simulink model "DC_Microgrid_Protection"  (R2022a)
settings: Solver=ode4  StartTime=0.0  StopTime=10  FixedStep=0.01  RelTol=1e-3
settings Model: Creator=nivas  LastModifiedBy=nivas

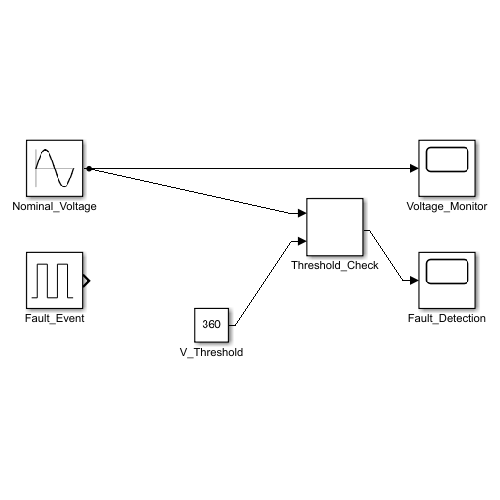
[thumbnail: Simulink's stored preview of the top-level diagram]
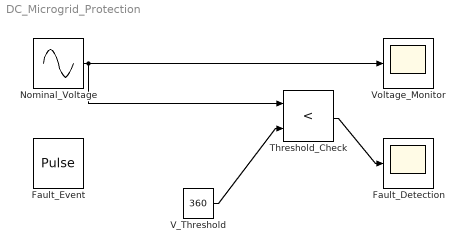
== system DC_Microgrid_Protection ==
  Fault_Detection : Scope
  Fault_Event : DiscretePulseGenerator  PulseType=Time based  Period=5  PulseWidth=20
  Nominal_Voltage : Sin  Amplitude=10  Bias=400  Frequency=0.5  SampleTime=0
  Threshold_Check : RelationalOperator  Operator=<  OutDataTypeStr=boolean  RndMeth=Simplest  InputSameDT=off
  V_Threshold : Constant  Value=360
  Voltage_Monitor : Scope
  wires:
  Nominal_Voltage/1 -> Voltage_Monitor/1, Threshold_Check/1
  V_Threshold/1 -> Threshold_Check/2
  Threshold_Check/1 -> Fault_Detection/1
